simulink library "phasedenvlib"  (R2015a)
settings: Solver=ode45  StartTime=0.0  StopTime=10.0  RelTol=1e-3
undefined symbols (not defined in the file or in its folder): phased, physconst
settings Model: CovSFcnEnable=off  Creator=The MathWorks Inc.  LastModifiedBy=The MathWorks Inc.
settings DebuggingCC: UnderspecifiedInitializationDetection=Classic  MergeDetectMultiDrivingBlocksExec=none  SolverPrmCheckMsg=warning

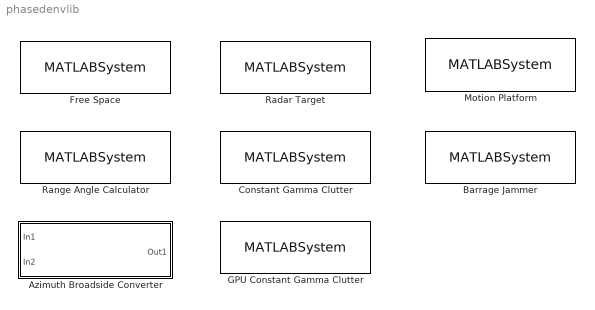
== system phasedenvlib ==
  Azimuth Broadside Converter : Subsystem  Variant=on  OverrideUsingVariant=AzimuthToBroadside  mask(Azimuth/broadside converter){Mode=azimuth -> broadside}
      mask prompts: Mode "Conversion mode:"
      mask help: Conversion between azimuth and broadside angles.
      mask init:
      | modestr = get_param(gcb,'Mode');
      | if modestr(1) == 'a'
      |     mvarctrl = 'AzimuthToBroadside';
      |     inportlabel = 'az';
      |     outportlabel = 'bsd';
      |     titlestr = 'az->bsd';
      | else
      |     mvarctrl = 'BroadsideToAzimuth';
      |     inportlabel = 'bsd';
      |     outportlabel = 'az';
      |     titlestr = 'bsd->az';
      | end
      | set_param(gcb, 'OverrideUsingVariant', mvarctrl);
      mask TypeOptions Mode: azimuth -> broadside | broadside -> azimuth
      mask Display:
      | port_label('input',1,inportlabel);
      | port_label('input',2,'el');
      | port_label('output',1,outportlabel);
      | fprintf('%s',titlestr)
  Barrage Jammer : MATLABSystem  System=phased.BarrageJammer  ERP=5000  SamplesPerFrameSource=Property  SamplesPerFrame=100  SeedSource=Property  Seed=randi(65535,1)  SimulateUsing=Interpreted execution
      mask Type: phased.BarrageJammer
      mask Display: disp('Barrage');
  Constant Gamma Clutter : MATLABSystem  System=phased.ConstantGammaClutter  Gamma=0  EarthModel=Flat  MaximumRange=5000  AzimuthCoverage=60  PatchAzimuthWidth=1  CoherenceTime=inf  PropagationSpeed=physconst( 'LightSpeed' )  SampleRate=1e6  PRF=1e4  OutputFormat=Pulses  NumPulses=1  NumSamples=100  OperatingFrequency=3e8  TransmitSignalInputPort=off  TransmitERP=5000  PlatformHeight=300  PlatformSpeed=300  PlatformDirection=[ 90; 0 ]  BroadsideDepressionAngle=0  SeedSource=Property  Seed=randi(65535,1)  Sensor=phased.ULA('Element',phased.IsotropicAntennaElement)  SimulateUsing=Interpreted execution
      mask Type: phased.ConstantGammaClutter
      mask Display: disp(['Constant' char(10) 'Gamma Clutter']);
  Free Space : MATLABSystem  System=phased.FreeSpace  PropagationSpeed=physconst( 'LightSpeed' )  OperatingFrequency=3e8  TwoWayPropagation=off  MaximumDistanceSource=Property  MaximumDistance=10e3  SimulateUsing=Interpreted execution
      mask Type: phased.FreeSpace
      mask Display:
      | disp(['Free Space' char(10) 'Channel']);
      | port_label('input',1,'X');
      | port_label('input',2,'Pos1');
      | port_label('input',3,'Pos2');
      | port_label('input',4,'Vel1');
      | port_label('input',5,'Vel2');
  GPU Constant Gamma Clutter : MATLABSystem  System=phased.gpu.ConstantGammaClutter  Gamma=0  EarthModel=Flat  MaximumRange=5000  AzimuthCoverage=60  PatchAzimuthWidth=1  CoherenceTime=inf  PropagationSpeed=physconst( 'LightSpeed' )  SampleRate=1e6  PRF=1e4  OutputFormat=Pulses  NumPulses=1  NumSamples=100  OperatingFrequency=3e8  TransmitSignalInputPort=off  TransmitERP=5000  PlatformHeight=300  PlatformSpeed=300  PlatformDirection=[ 90; 0 ]  BroadsideDepressionAngle=0  SeedSource=Auto  Seed=0  Sensor=phased.ULA('Element',phased.IsotropicAntennaElement)  SimulateUsing=Interpreted execution
      mask Type: phased.gpu.ConstantGammaClutter
      mask Display: disp(['GPU Constant' char(10) 'Gamma Clutter']);
  Motion Platform : MATLABSystem  System=phased.Platform  InitialPosition=[ 0; 0; 0 ]  Velocity=[ 0; 0; 0 ]  OrientationAxes=eye( 3 )  OrientationAxesOutputPort=off  SimulateUsing=Interpreted execution
      mask Type: phased.Platform
      mask Display:
      | disp('Platform');
      | port_label('output',1,'Pos');
      | port_label('output',2,'Vel');
  Radar Target : MATLABSystem  System=phased.RadarTarget  EnablePolarization=off  Mode=Monostatic  MeanRCSSource=Property  ScatteringMatrixSource=Property  MeanRCS=1  ScatteringMatrix=eye( 2 )  Model=Nonfluctuating  PropagationSpeed=physconst( 'LightSpeed' )  OperatingFrequency=3e8  SeedSource=Property  Seed=randi(65535,1)  SimulateUsing=Interpreted execution
      mask Type: phased.RadarTarget
      mask Display:
      | disp('Target');
      | port_label('input',1,'X');
  Range Angle Calculator : MATLABSystem  System=phased.internal.RangeAngle  ReferencePositionSource=Property  ReferencePosition=[ 0; 0; 0 ]  ReferenceAxesSource=Property  ReferenceAxes=eye( 3 )  Output=Angle  SimulateUsing=Interpreted execution
      mask Type: phased.internal.RangeAngle
      mask Display:
      | disp(['Range' char(10) 'Angle']);
      | port_label('input',1,'Pos');
      | port_label('output',1,'Ang');

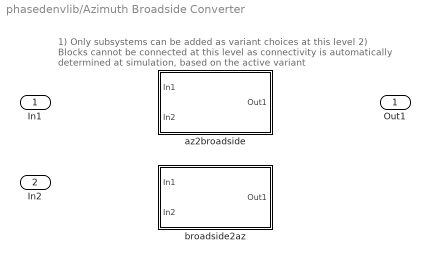
== system phasedenvlib/Azimuth Broadside Converter ==
  note: 1) Only subsystems can be added as variant choices at this level
      | 2) Blocks cannot be connected at this level as connectivity is
      | automatically determined at simulation, based on the active variant
  In1 : Inport
  In2 : Inport  Port=2
  az2broadside : Subsystem  VariantControl=AzimuthToBroadside
  broadside2az : Subsystem  VariantControl=BroadsideToAzimuth
  Out1 : Outport

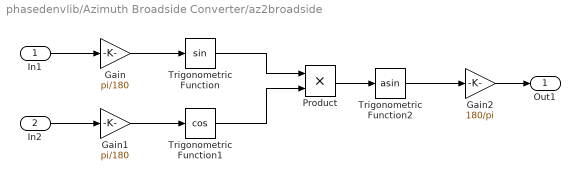
== system phasedenvlib/Azimuth Broadside Converter/az2broadside ==
  In1 : Inport
  In2 : Inport  Port=2
  Gain : Gain  Gain=pi/180
  Gain1 : Gain  Gain=pi/180
  Gain2 : Gain  Gain=180/pi
  Product : Product
  Trigonometric Function : Trigonometry
  Trigonometric Function1 : Trigonometry  Operator=cos
  Trigonometric Function2 : Trigonometry  Operator=asin
  Out1 : Outport
  wires:
  Product/1 -> Trigonometric Function2/1
  Gain2/1 -> Out1/1
  Trigonometric Function1/1 -> Product/2
  Trigonometric Function/1 -> Product/1
  Trigonometric Function2/1 -> Gain2/1
  Gain/1 -> Trigonometric Function/1
  In1/1 -> Gain/1
  In2/1 -> Gain1/1
  Gain1/1 -> Trigonometric Function1/1

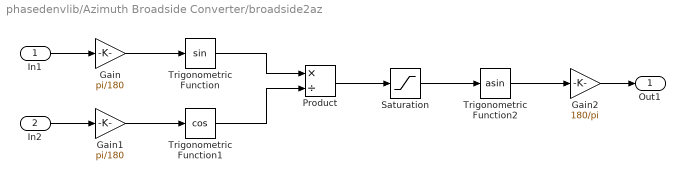
== system phasedenvlib/Azimuth Broadside Converter/broadside2az ==
  In1 : Inport
  In2 : Inport  Port=2
  Gain : Gain  Gain=pi/180
  Gain1 : Gain  Gain=pi/180
  Gain2 : Gain  Gain=180/pi
  Product : Product  Inputs=*/
  Saturation : Saturate  UpperLimit=1  LowerLimit=-1
  Trigonometric Function : Trigonometry
  Trigonometric Function1 : Trigonometry  Operator=cos
  Trigonometric Function2 : Trigonometry  Operator=asin
  Out1 : Outport
  wires:
  Saturation/1 -> Trigonometric Function2/1
  Gain1/1 -> Trigonometric Function1/1
  In2/1 -> Gain1/1
  In1/1 -> Gain/1
  Gain/1 -> Trigonometric Function/1
  Trigonometric Function2/1 -> Gain2/1
  Trigonometric Function/1 -> Product/1
  Trigonometric Function1/1 -> Product/2
  Gain2/1 -> Out1/1
  Product/1 -> Saturation/1
